simulink model "MIL_Visualisation"  (R2022b)
settings: Solver=VariableStepAuto  StartTime=0.0  StopTime=60  RelTol=1e-3
libraries: slpidlib x2, sim3dlib x1, sim3dautolib x1
settings Model: Creator=ok  LastModifiedBy=ok

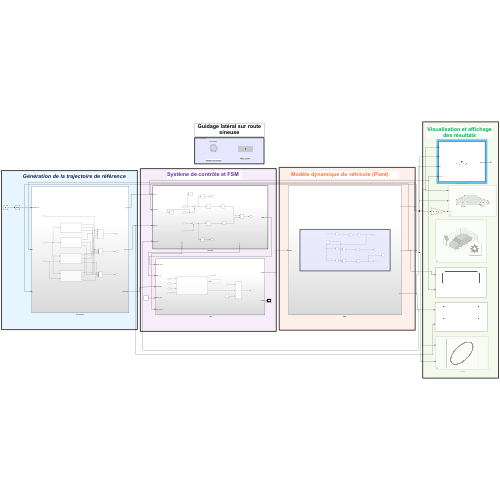
[thumbnail: Simulink's stored preview of the top-level diagram]
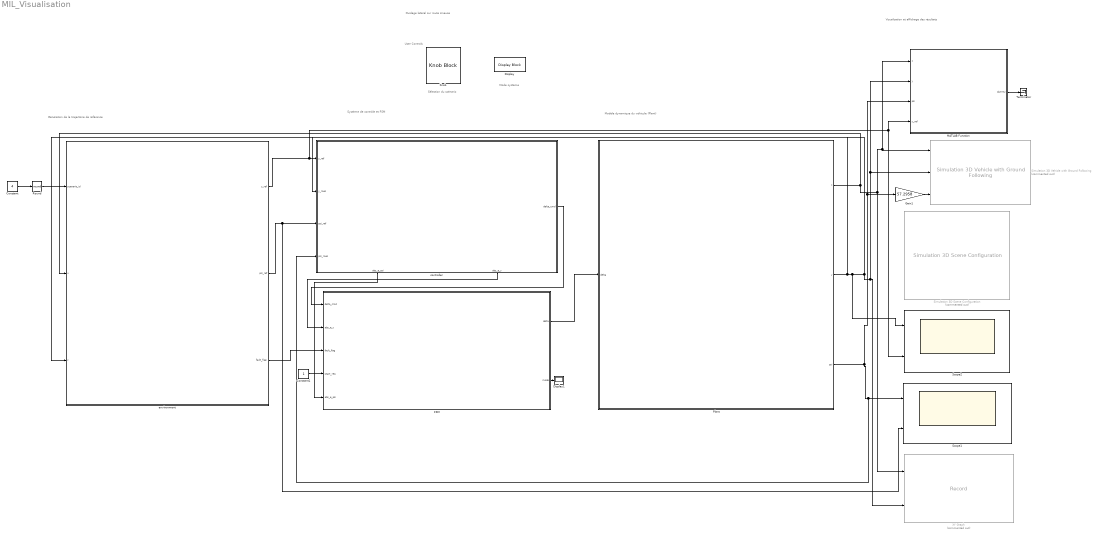
== system MIL_Visualisation ==
  note: Système de contrôle et FSM
  note: Génération de la trajectoire de référence
  note: Visualisation et affichage des résultats
  note: Sélection du scénario
  note: Mode système
  note: User Controls
  note: Modèle dynamique du véhicule (Plant)
  note: Guidage latéral sur route sineuse
  Constant : Constant  Value=4
  Constant1 : Constant
  Display : DisplayBlock  LabelPosition=Hide  Transparency=1
  Display1 : Display
  FSM : Subsystem
  Gain1 : Gain  Gain=57.2958
  Knob : KnobBlock  ScaleMin=1  ScaleMax=4  TickInterval=1
  MATLAB Function : MATLAB Function  TreatAsAtomicUnit=on
  "Plant " : Subsystem
  Round : Rounding  Operator=round
  Scope1 : Scope  NumInputPorts=2
  Scope2 : Scope  NumInputPorts=2
  Simulation 3D Scene Configuration : sim3dlib/Simulation 3D Scene Configuration  Priority=0  Commented=on  ProjectFormat=Default Scenes  SceneDesc=Straight road  ProjectName=C:\Program Files\MATLAB\R2022b\toolbox\shared\sim3d_projects\automotive_project\UE4\WindowsNoEditor\VehicleSimulation.exe  ScenePath=/Game/Maps/HwStrght  EnableOpenDRIVE=off  vehTagList={'Scene Origin';'SimulinkVehicle1'}  vehTag=Scene Origin  OpVisEn=off  Ts=1/60  EnableWindow=on  EnableRemoteAccess=off  EnableWeather=off  SunAltitude=40.0  SunAzimuth=90  clouds=10  wind=1  fog=0  rain=0  EnableGeospatial=off  OriginHeight=200  OriginLatitude=40.744652  OriginLongitude=-73.988864  MapStyle=Aerial  AdditionalAssetIDs=[]  UseAdvancedSunSky=off  SolarTime=11  TimeZone=-5  Day=21  Month=9  Year=2022  UseDaylightSavingTime=on  DSTStartDay=10  DSTStartMonth=3  DSTEndDay=3  DSTEndMonth=11  DSTSwitchHour=2  sensorTag=MainCamera1  sensorId=1  sensorName=MainCamera1  mountLoc=Origin  offsetFlag=off  tmountOffset=[0, 0, 0]  rmountOffset=[0, 0, 0]  HorizontalResolution=1280  VerticalResolution=720  HorizontalFOV=60  mountPoint=[0 0 0]  mountOrientation=[0 0 0]  aMode=3  ID=1  GeoTrigger=Inactive
      settings: LibrarySourceBlock=drivingsim3d/Simulation 3D Scene Configuration
  Simulation 3D Vehicle with Ground Following : sim3dautolib/Simulation 3D Vehicle with Ground Following  Priority=-1  Commented=on  PassVehMesh=Muscle car  MeshPath=/MathWorksAutomotiveContent/Vehicles/Muscle/Meshes/SK_MuscleCar.SK_MuscleCar  TrackWidth=1.9  WheelBase=3  WheelRadius=0.35  VehColor=Orange  InitialPos=[0, 0, 0]  InitialRot=[0, 0, 0]  ActorName=SimulinkVehicle1  SampleTime=-1  ActorType=SimulinkVehicle  ID=1  aMode=3  ActorTag=SimulinkVehicle1  CoordinateScheme=ISO  VehLightsControl=off  HeadlightColor=[ 1, 1, 1 ]  HighBeamIntensity=100000  LowBeamIntensity=60000  HighBeamConeAngle=70  LowBeamConeAngle=70  LeftHeadlightOrientation=[ 0, 0 ]  RightHeadlightOrientation=[ 0, 0 ]  BrakelightIntensity=500  ReverselightIntensity=500  SignallightIntensity=500  SignallightPeriod=1  SignalPulseWidth=50  TransformOutportEnabled=off
      settings: LibrarySourceBlock=drivingsim3d/Simulation 3D Vehicle with Ground Following
  Terminator : Terminator
  XY Graph : Record  Commented=on  FileSettingsInternal="{\"entries\":[{\"content\":{\"excelSettings\":{\"content\":{},\"type\":\"Streamout.ExcelSettings\"}},\"type\":\"Streamout.FileSettingStorage\",\"uuid\":\"06e8999a-84d6-4fbe-90db-6198f86497ce\"}],\"packageUris\":[\"http://schema.mathworks.com/mf0/streamout_blocks/R2020a\"],\"version\":\"1.0\"}"  Layout=[1 1]  SignalsInternal="{\"entries\":[{\"content\":{\"signals\":[{\"content\":{\"blockPath\":[\"testMIL/XY Graph\"],\"channel\":[],\"dimensions\":[1],\"domain\":\"testMIL/XY Graph\",\"lineColor\":\"#edb120\",\"plots\":[],\"port\":1,\"sid\":[],\"signalID\":1014,\"signalName\":\"Plant :1\"},\"type\":\"RecordBlkView.Signal\",\"uuid\":\"2eb3453d-083d-4465-a58f-0ec1d1455d5e\"},{\"content\":{\"blockPath\":[\"testMIL/XY Graph\"],\"channel\":[],\"dimensions\":[1],\"domain\":\"testMIL/XY Graph\",\"lineColor\":\"#7e2f8e\",\"plots\":[],\"port\":2,\"sid\":[],\"signalID\":1017,\"signalName\":\"Plant :2\"},\"type\":\"RecordBlkView.Signal\",\"uuid\":\"a053f1bc-5d23-4c0a-8de6-d9fee1b0b9c1\"}]},\"type\":\"RecordBlkView.InputSignals\",\"uuid\":\"f97cfab6-83bd-41ff-8d9c-43b8d98c9b4b\"}],\"packageUris\":[\"http://schema.mathworks.com/mf0/streamout_blocks/R2020a\"],\"version\":\"1.0\"}"  VisualizationBindings="{\"xyplotplugin\":{\"info\":[{\"series\":[],\"subplotID\":1}]}}"  CompatibilityTag=XY
  controller : Subsystem  TreatAsAtomicUnit=on
      settings: PortSchema="{\"entries\":[{\"content\":{\"sides\":[{\"content\":{\"connectorIds\":[\"In1\",\"In2\",\"In3\",\"In4\"]},\"type\":\"ConnectorPlacement.EquallySpacedRectSide\",\"uuid\":\"dce009df-b000-45c7-aa28-a3bb8a55b1fe\"},{\"content\":{\"connectorIds\":[\"Out1\"],\"side\":\"RIGHT\"},\"type\":\"ConnectorPlacement.EquallySpacedRectSide\",\"uuid\":\"27679ab1-5f7b-49ed-b0db-4270332b706f\"},{\"content\":{\"connectorIds\":[],\"side\":\"TOP\"},\"type\":\"ConnectorPlacement.EquallySpacedRectSide\",\"uuid\":\"474e0d2f-310b-4a94-af54-f468ed9e1b68\"},{\"content\":{\"connectorIds\":[\"Out2\",\"Out3\"],\"side\":\"BOTTOM\"},\"type\":\"ConnectorPlacement.EquallySpacedRectSide\",\"uuid\":\"e9194f37-6c87-4243-879e-6146eac92453\"}]},\"type\":\"ConnectorPlacement.EquallySpacedConnector\",\"uuid\":\"bf9faa3f-a673-4ccc-8b0a-d91001fa1506\"}],\"packageUris\":[\"http://schema.mathworks.com/mf0/Connector/R2020b\"],\"version\":\"1.0\"}"
  "environment " : Subsystem
  wires:
  "Plant "/1(x) -> XY Graph/1, Simulation 3D Vehicle with Ground Following/1, MATLAB Function/1(x), "environment "/2(x)
  controller/3(abs_e_y) -> FSM/2(abs_e_y)
  controller/2(abs_e_psi) -> FSM/5(abs_e_psi)
  "environment "/3(fault_flag) -> FSM/3(fault_flag)
  FSM/2(mode) -> Display1/1
  Constant/1 -> Round/1
  "Plant "/3(psi) -> controller/4(psi_mes), Scope1/1, Gain1/1, MATLAB Function/3(psi)
  "environment "/2(psi_ref) -> Scope1/2, controller/3(psi_ref)
  Round/1 -> "environment "/1(scenario_id)
  Constant1/1 -> FSM/4(start_req)
  FSM/1(delta) -> "Plant "/1(delta)
  "environment "/1(y_ref) -> MATLAB Function/4(y_ref), Scope2/2, controller/1(y_ref)
  MATLAB Function/1(dummy) -> Terminator/1
  "Plant "/2(y) -> controller/2(y_mes), Scope2/1, XY Graph/2, MATLAB Function/2(y), Simulation 3D Vehicle with Ground Following/2, "environment "/3(y)
  controller/1(delta_cmd) -> FSM/1(delta_cmd)
  Gain1/1 -> Simulation 3D Vehicle with Ground Following/3

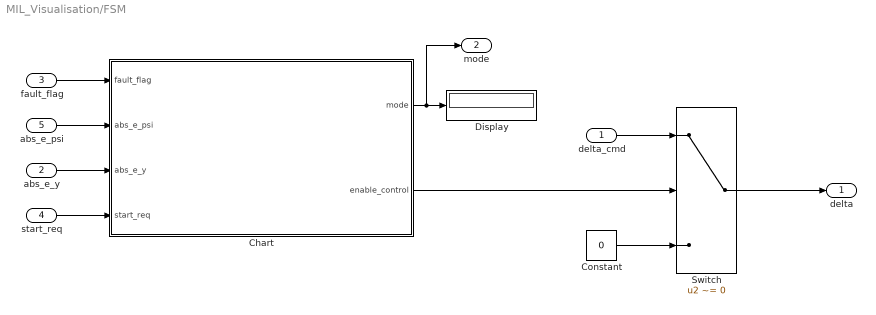
== system MIL_Visualisation/FSM ==
  delta_cmd : Inport
  abs_e_y : Inport  Port=2
  fault_flag : Inport  Port=3
  start_req : Inport  Port=4
  abs_e_psi : Inport  Port=5
  Chart : Stateflow chart  TreatAsAtomicUnit=on
  Constant : Constant  Value=0
  Display : Display
  Switch : Switch  Criteria=u2 ~= 0  SaturateOnIntegerOverflow=off  InputSameDT=off
  delta : Outport
  mode : Outport  Port=2
  wires:
  Chart/1(mode) -> mode/1, Display/1
  delta_cmd/1 -> Switch/1
  Switch/1 -> delta/1
  Chart/2(enable_control) -> Switch/2
  Constant/1 -> Switch/3
  abs_e_y/1 -> Chart/3(abs_e_y)
  fault_flag/1 -> Chart/1(fault_flag)
  abs_e_psi/1 -> Chart/2(abs_e_psi)
  start_req/1 -> Chart/4(start_req)

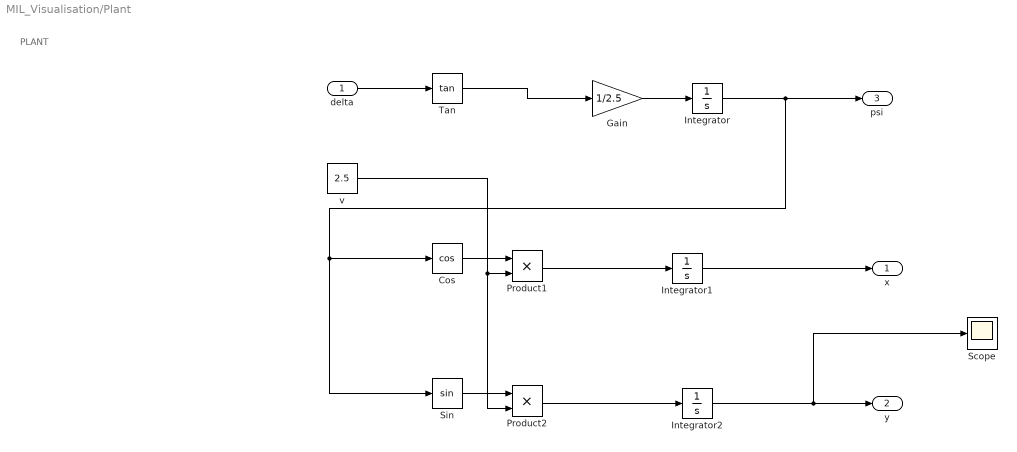
== system MIL_Visualisation/Plant  ==
  note: PLANT
  delta : Inport
  Cos : Trigonometry  Operator=cos
  Gain : Gain  Gain=1/2.5
  Integrator : Integrator
  Integrator1 : Integrator
  Integrator2 : Integrator
  Product1 : Product
  Product2 : Product
  Scope : Scope
  Sin : Trigonometry
  Tan : Trigonometry  Operator=tan
  v : Constant  Value=2.5
  x : Outport
  y : Outport  Port=2
  psi : Outport  Port=3
  wires:
  delta/1 -> Tan/1
  v/1 -> Product2/2, Product1/2
  Gain/1 -> Integrator/1
  Integrator/1 -> Sin/1, Cos/1, psi/1
  Cos/1 -> Product1/1
  Product1/1 -> Integrator1/1
  Integrator1/1 -> x/1
  Sin/1 -> Product2/1
  Product2/1 -> Integrator2/1
  Integrator2/1 -> Scope/1, y/1
  Tan/1 -> Gain/1

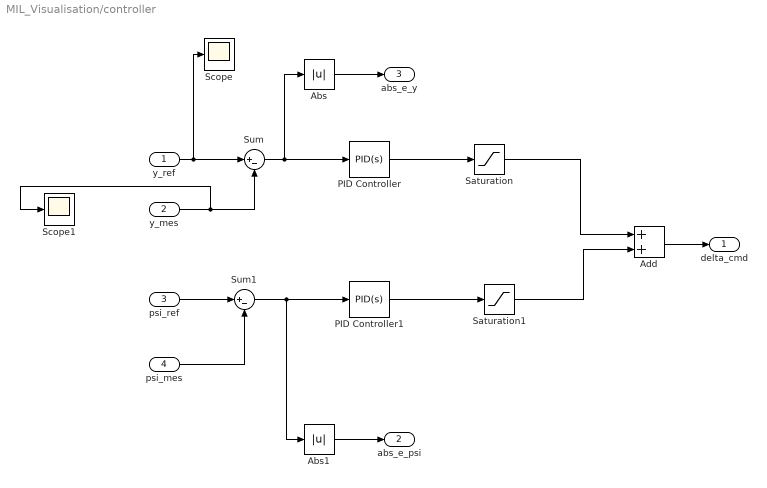
== system MIL_Visualisation/controller ==
  y_ref : Inport
  y_mes : Inport  Port=2
  psi_ref : Inport  Port=3
  psi_mes : Inport  Port=4
  Abs : Abs  SaturateOnIntegerOverflow=off
  Abs1 : Abs  SaturateOnIntegerOverflow=off
  Add : Sum
  PID Controller : slpidlib/PID Controller  Controller=PID  Form=Parallel  TimeDomain=Continuous-time  UseExternalTs=off  SampleTime=-1  IntegratorMethod=Forward Euler  FilterMethod=Forward Euler  ControllerParametersSource=internal  P=0.543076883773547  I=0.448698988285461  UseKiTs=off  D=0.162626525747815  N=212.929749678129  UseFilter=on  TunerSelectOption=Transfer Function Based (PID Tuner App)  InitialConditionSource=internal  InitialConditionForIntegrator=0  InitialConditionForFilter=0  DifferentiatorICPrevScaledInput=0  ExternalReset=none  TrackingMode=off  Kt=1  LimitOutput=off  SatLimitsSource=internal  UpperSaturationLimit=inf  LowerSaturationLimit=-inf  LinearizeAsGain=on  AntiWindupMode=none  Kb=1  LimitIntegrator=off  UpperIntegratorSaturationLimit=inf  LowerIntegratorSaturationLimit=-inf  POutMin=[]  POutMax=[]  IOutMin=[]  IOutMax=[]  DOutMin=[]  DOutMax=[]  NOutMin=[]  NOutMax=[]  SumOutMin=[]  SumOutMax=[]  SaturationOutMin=[]  SaturationOutMax=[]  PParamMin=[]  PParamMax=[]  IParamMin=[]  IParamMax=[]  DParamMin=[]  DParamMax=[]  NParamMin=[]  NParamMax=[]  KbParamMin=[]  KbParamMax=[]  KtParamMin=[]  KtParamMax=[]  KbOutMin=[]  KbOutMax=[]  KtOutMin=[]  KtOutMax=[]  IntegratorOutMin=[]  IntegratorOutMax=[]  FilterOutMin=[]  FilterOutMax=[]  SumI1OutMin=[]  SumI1OutMax=[]  SumI2OutMin=[]  SumI2OutMax=[]  SumI3OutMin=[]  SumI3OutMax=[]  SumI4OutMin=[]  SumI4OutMax=[]  SumDOutMin=[]  SumDOutMax=[]  DifferentiatorOutMin=[]  DifferentiatorOutMax=[]  FilterDiffOutCoefMin=[]  FilterDiffOutCoefMax=[]  ReciprocalOutMin=[]  ReciprocalOutMax=[]  SumDenOutMin=[]  SumDenOutMax=[]  SumNumOutMin=[]  SumNumOutMax=[]  DivideOutMin=[]  DivideOutMax=[]  UdiffTsProdOutMin=[]  UdiffTsProdOutMax=[]  NTsProdOutMin=[]  NTsProdOutMax=[]  UintegralTsProdOutMin=[]  UintegralTsProdOutMax=[]  UngainTsProdOutMin=[]  UngainTsProdOutMax=[]  ClampingZeroOutDataTypeStr=Inherit: Inherit via back propagation  ClampingZeroOutMin=[]  ClampingZeroOutMax=[]  FilterDenConstantOutDataTypeStr=Inherit: Inherit via back propagation  FilterDenConstantOutMin=[]  FilterDenConstantOutMax=[]  PCopyOutDataTypeStr=Inherit: Inherit via back propagation  PCopyOutMin=[]  PCopyOutMax=[]  NCopyOutDataTypeStr=Inherit: Inherit via back propagation  NCopyOutMin=[]  NCopyOutMax=[]  IntegratorContinuousStateAttributes=''  IntegratorStateMustResolveToSignalObject=off  IntegratorRTWStateStorageClass=Auto  FilterContinuousStateAttributes=''  FilterStateMustResolveToSignalObject=off  FilterRTWStateStorageClass=Auto  ParallelPVariant=InternalParameters  IdealPVariant=Disabled  IVariant=InternalParameters  DVariant=InternalParameters  IntegratorVariant=Continuous  SatVariant=Disabled  AWVariant=Passthrough  PCopyVariant=Disabled  TRVariant=Disabled  FdbkBlocksVariant=Forward  IdealPFdbkVariant=Disabled  SatFdbkVariant=Disabled  DerivativeFilterVariant=ContFilter  NVariant=InternalParameters  NCopyVariant=Disabled  FilterICVariant=InternalICsFilter  IntegratorICVariant=InternalICs  ExternalResetVariant=Disabled  TRSumVariant=Passthrough  SumFdbkVariant=Disabled  SumVariant=Sum_PID  TsampFilterVariant=InternalTs  TsampNgainVariant=Passthrough  TsampIntegralVariant=Passthrough  ExternalSaturationOutDataTypeStr=Inherit: Same as second input
  PID Controller1 : slpidlib/PID Controller  Controller=PID  Form=Parallel  TimeDomain=Continuous-time  UseExternalTs=off  SampleTime=-1  IntegratorMethod=Forward Euler  FilterMethod=Forward Euler  ControllerParametersSource=internal  P=68.8464008350311  I=1387.43622401745  UseKiTs=off  D=-0.169418101050233  N=123.850290878266  UseFilter=on  TunerSelectOption=Transfer Function Based (PID Tuner App)  InitialConditionSource=internal  InitialConditionForIntegrator=0  InitialConditionForFilter=0  DifferentiatorICPrevScaledInput=0  ExternalReset=none  TrackingMode=off  Kt=1  LimitOutput=off  SatLimitsSource=internal  UpperSaturationLimit=inf  LowerSaturationLimit=-inf  LinearizeAsGain=on  AntiWindupMode=none  Kb=1  LimitIntegrator=off  UpperIntegratorSaturationLimit=inf  LowerIntegratorSaturationLimit=-inf  POutMin=[]  POutMax=[]  IOutMin=[]  IOutMax=[]  DOutMin=[]  DOutMax=[]  NOutMin=[]  NOutMax=[]  SumOutMin=[]  SumOutMax=[]  SaturationOutMin=[]  SaturationOutMax=[]  PParamMin=[]  PParamMax=[]  IParamMin=[]  IParamMax=[]  DParamMin=[]  DParamMax=[]  NParamMin=[]  NParamMax=[]  KbParamMin=[]  KbParamMax=[]  KtParamMin=[]  KtParamMax=[]  KbOutMin=[]  KbOutMax=[]  KtOutMin=[]  KtOutMax=[]  IntegratorOutMin=[]  IntegratorOutMax=[]  FilterOutMin=[]  FilterOutMax=[]  SumI1OutMin=[]  SumI1OutMax=[]  SumI2OutMin=[]  SumI2OutMax=[]  SumI3OutMin=[]  SumI3OutMax=[]  SumI4OutMin=[]  SumI4OutMax=[]  SumDOutMin=[]  SumDOutMax=[]  DifferentiatorOutMin=[]  DifferentiatorOutMax=[]  FilterDiffOutCoefMin=[]  FilterDiffOutCoefMax=[]  ReciprocalOutMin=[]  ReciprocalOutMax=[]  SumDenOutMin=[]  SumDenOutMax=[]  SumNumOutMin=[]  SumNumOutMax=[]  DivideOutMin=[]  DivideOutMax=[]  UdiffTsProdOutMin=[]  UdiffTsProdOutMax=[]  NTsProdOutMin=[]  NTsProdOutMax=[]  UintegralTsProdOutMin=[]  UintegralTsProdOutMax=[]  UngainTsProdOutMin=[]  UngainTsProdOutMax=[]  ClampingZeroOutDataTypeStr=Inherit: Inherit via back propagation  ClampingZeroOutMin=[]  ClampingZeroOutMax=[]  FilterDenConstantOutDataTypeStr=Inherit: Inherit via back propagation  FilterDenConstantOutMin=[]  FilterDenConstantOutMax=[]  PCopyOutDataTypeStr=Inherit: Inherit via back propagation  PCopyOutMin=[]  PCopyOutMax=[]  NCopyOutDataTypeStr=Inherit: Inherit via back propagation  NCopyOutMin=[]  NCopyOutMax=[]  IntegratorContinuousStateAttributes=''  IntegratorStateMustResolveToSignalObject=off  IntegratorRTWStateStorageClass=Auto  FilterContinuousStateAttributes=''  FilterStateMustResolveToSignalObject=off  FilterRTWStateStorageClass=Auto  ParallelPVariant=InternalParameters  IdealPVariant=Disabled  IVariant=InternalParameters  DVariant=InternalParameters  IntegratorVariant=Continuous  SatVariant=Disabled  AWVariant=Passthrough  PCopyVariant=Disabled  TRVariant=Disabled  FdbkBlocksVariant=Forward  IdealPFdbkVariant=Disabled  SatFdbkVariant=Disabled  DerivativeFilterVariant=ContFilter  NVariant=InternalParameters  NCopyVariant=Disabled  FilterICVariant=InternalICsFilter  IntegratorICVariant=InternalICs  ExternalResetVariant=Disabled  TRSumVariant=Passthrough  SumFdbkVariant=Disabled  SumVariant=Sum_PID  TsampFilterVariant=InternalTs  TsampNgainVariant=Passthrough  TsampIntegralVariant=Passthrough  ExternalSaturationOutDataTypeStr=Inherit: Same as second input
  Saturation : Saturate
  Saturation1 : Saturate
  Scope : Scope
  Scope1 : Scope
  Sum : Sum  Inputs=|+-
  Sum1 : Sum  Inputs=|+-
  delta_cmd : Outport
  abs_e_psi : Outport  Port=2
  abs_e_y : Outport  Port=3
  wires:
  y_ref/1 -> Scope/1, Sum/1
  y_mes/1 -> Scope1/1, Sum/2
  Sum/1 -> PID Controller/1, Abs/1
  psi_ref/1 -> Sum1/1
  psi_mes/1 -> Sum1/2
  PID Controller/1 -> Saturation/1
  Sum1/1 -> Abs1/1, PID Controller1/1
  PID Controller1/1 -> Saturation1/1
  Add/1 -> delta_cmd/1
  Saturation/1 -> Add/1
  Saturation1/1 -> Add/2
  Abs/1 -> abs_e_y/1
  Abs1/1 -> abs_e_psi/1

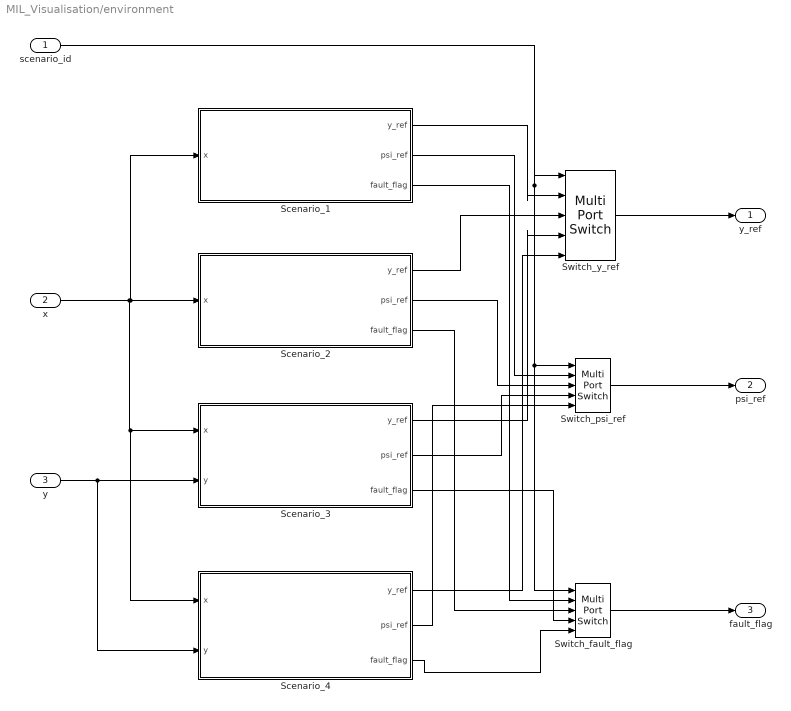
== system MIL_Visualisation/environment  ==
  scenario_id : Inport
  x : Inport  Port=2
  y : Inport  Port=3
  Scenario_1 : Subsystem
  Scenario_2 : Subsystem
  Scenario_3 : Subsystem
  Scenario_4 : Subsystem
  Switch_fault_flag : MultiPortSwitch  Inputs=4  SaturateOnIntegerOverflow=off  InputSameDT=off
  Switch_psi_ref : MultiPortSwitch  Inputs=4  SaturateOnIntegerOverflow=off  InputSameDT=off
  Switch_y_ref : MultiPortSwitch  Inputs=4  SaturateOnIntegerOverflow=off  InputSameDT=off
  y_ref : Outport
  psi_ref : Outport  Port=2
  fault_flag : Outport  Port=3
  wires:
  scenario_id/1 -> Switch_fault_flag/1, Switch_psi_ref/1, Switch_y_ref/1
  Scenario_1/1(y_ref) -> Switch_y_ref/2
  Scenario_2/1("y_ref ") -> Switch_y_ref/3
  Scenario_3/1("y_ref ") -> Switch_y_ref/4
  Scenario_4/1(y_ref) -> Switch_y_ref/5
  Scenario_1/2(psi_ref) -> Switch_psi_ref/2
  Scenario_2/2("psi_ref ") -> Switch_psi_ref/3
  Scenario_3/2("psi_ref ") -> Switch_psi_ref/4
  Scenario_4/2(psi_ref) -> Switch_psi_ref/5
  Scenario_1/3(fault_flag) -> Switch_fault_flag/2
  Scenario_2/3(fault_flag) -> Switch_fault_flag/3
  Scenario_3/3(fault_flag) -> Switch_fault_flag/4
  Scenario_4/3(fault_flag) -> Switch_fault_flag/5
  Switch_fault_flag/1 -> fault_flag/1
  Switch_psi_ref/1 -> psi_ref/1
  Switch_y_ref/1 -> y_ref/1
  x/1 -> Scenario_4/1(x), Scenario_3/1(x), Scenario_1/1(x), Scenario_2/1(x)
  y/1 -> Scenario_4/2(y), Scenario_3/2(y)

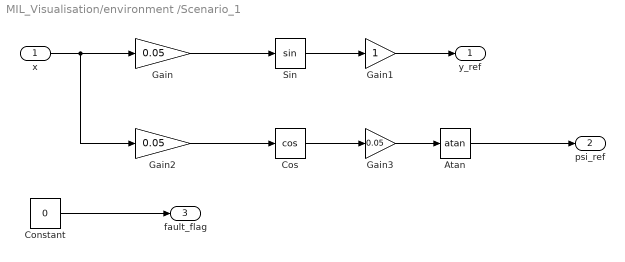
== system MIL_Visualisation/environment /Scenario_1 ==
  x : Inport
  Atan : Trigonometry  Operator=atan
  Constant : Constant  Value=0
  Cos : Trigonometry  Operator=cos
  Gain : Gain  Gain=0.05
  Gain1 : Gain
  Gain2 : Gain  Gain=0.05
  Gain3 : Gain  Gain=0.05
  Sin : Trigonometry
  y_ref : Outport
  psi_ref : Outport  Port=2
  fault_flag : Outport  Port=3
  wires:
  x/1 -> Gain2/1, Gain/1
  Gain/1 -> Sin/1
  Sin/1 -> Gain1/1
  Gain1/1 -> y_ref/1
  Cos/1 -> Gain3/1
  Gain2/1 -> Cos/1
  Gain3/1 -> Atan/1
  Atan/1 -> psi_ref/1
  Constant/1 -> fault_flag/1

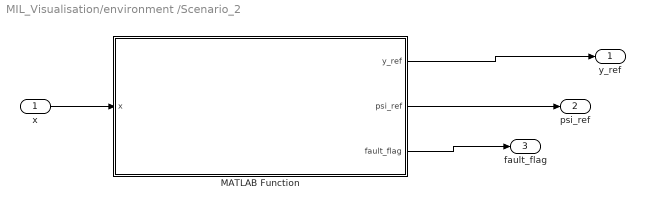
== system MIL_Visualisation/environment /Scenario_2 ==
  x : Inport
  MATLAB Function : MATLAB Function  TreatAsAtomicUnit=on
  "y_ref " : Outport
  "psi_ref " : Outport  Port=2
  fault_flag : Outport  Port=3
  wires:
  MATLAB Function/1(y_ref) -> "y_ref "/1
  MATLAB Function/2(psi_ref) -> "psi_ref "/1
  MATLAB Function/3(fault_flag) -> fault_flag/1
  x/1 -> MATLAB Function/1(x)

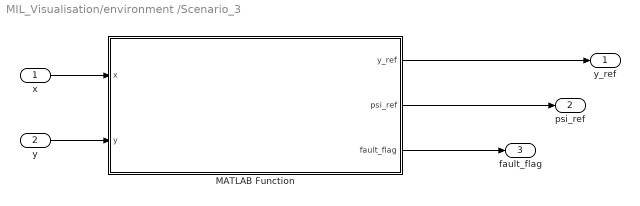
== system MIL_Visualisation/environment /Scenario_3 ==
  x : Inport
  y : Inport  Port=2
  MATLAB Function : MATLAB Function  TreatAsAtomicUnit=on
  "y_ref " : Outport
  "psi_ref " : Outport  Port=2
  fault_flag : Outport  Port=3
  wires:
  MATLAB Function/1(y_ref) -> "y_ref "/1
  MATLAB Function/3(fault_flag) -> fault_flag/1
  y/1 -> MATLAB Function/2(y)
  MATLAB Function/2(psi_ref) -> "psi_ref "/1
  x/1 -> MATLAB Function/1(x)

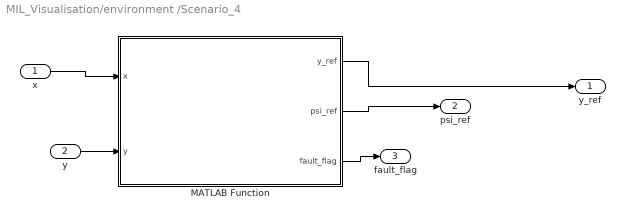
== system MIL_Visualisation/environment /Scenario_4 ==
  x : Inport
  y : Inport  Port=2
  MATLAB Function : MATLAB Function  TreatAsAtomicUnit=on
  y_ref : Outport
  psi_ref : Outport  Port=2
  fault_flag : Outport  Port=3
  wires:
  x/1 -> MATLAB Function/1(x)
  MATLAB Function/1(y_ref) -> y_ref/1
  MATLAB Function/2(psi_ref) -> psi_ref/1
  MATLAB Function/3(fault_flag) -> fault_flag/1
  y/1 -> MATLAB Function/2(y)

== matlab function MIL_Visualisation/environment /Scenario_3/MATLAB Function ==
  data: x input; y_ref output; y input; psi_ref output; fault_flag output
function [y_ref, psi_ref, fault_flag] = scenario3_onecurve(x, y)
%#codegen

% Paramètres de la route
A = 2.0;      % amplitude de la courbe
xc = 25.0;    % centre de la courbe
sigma = 6.0;  % largeur de la courbe

% Référence latérale : une seule bosse douce
dx = x - xc;
y_ref = A * exp(-(dx*dx)/(2*sigma*sigma));

% Dérivée par rapport à x
dy_dx = y_ref * ( -dx / (sigma*sigma) );

% Orientation de référence
psi_ref = atan(dy_dx);

% Pas de défaut dans ce scénario
fault_flag = 0;

== matlab function MIL_Visualisation/environment /Scenario_2/MATLAB Function ==
  data: x input; y_ref output; psi_ref output; fault_flag output
function [y_ref, psi_ref, fault_flag] = environment_fun(x)
%#codegen

% Route sinueuse simple et cohérente
A = 2;       % amplitude
B = 0.1;     % fréquence spatiale

y_ref = A*sin(B*x);

% pente de la route
dy_dx = A*B*cos(B*x);

% orientation de la route
psi_ref = atan(dy_dx);

% défaut
fault_flag = 0;

end

== stateflow chart MIL_Visualisation/FSM/Chart ==
  state Init
    en:
    enable_control = 0;
    mode = 0;
  state Nominal
    en:
    enable_control = 1;
    mode = 2;
  state Standby
    en:
    enable_control = 0;
    mode = 1;
  state Emergency
    en:
    enable_control = 0;
    mode = 3;
  (default) -> Init
  Standby -> Nominal : [start_req == 1 && fault_flag == 0]
  Init -> Standby : after(0.5,sec)
  Emergency -> Standby : [start_req == 0 && fault_flag == 0]
  Nominal -> Emergency : [fault_flag == 1 || abs_e_y > 1.5 || abs_e_psi > 0.5]
  data: mode output; enable_control output; fault_flag input; abs_e_psi input; abs_e_y input; start_req input

== matlab function MIL_Visualisation/MATLAB Function ==
  settings: updateMethod=DISCRETE
  data: x input; dummy output; y input; psi input; y_ref input
function dummy = draw_vehicle_2D(x, y, psi, y_ref)
%#codegen

coder.extrinsic('figure','clf','hold','grid','xlabel','ylabel', ...
                'title','legend','plot','fill','set','xlim','ylim', ...
                'drawnow','gca','gcf')

persistent hTraj hRef hCar Xveh Yveh Xref Yref isInit ax fig

dummy = 0;

if isempty(isInit)
    fig = figure(20);
    clf(fig);

    % Grande fenêtre
    set(fig,'Units','normalized');
    set(fig,'Position',[0.08 0.08 0.84 0.82]);

    ax = gca;
    hold(ax,'on');
    grid(ax,'on');

    % IMPORTANT : ne pas mettre axis equal
    set(ax,'Units','normalized');
    set(ax,'Position',[0.06 0.10 0.90 0.82]);

    xlabel(ax,'X [m]','FontSize',14);
    ylabel(ax,'Y [m]','FontSize',14);
    title(ax,'Suivi 2D du vehicule sur route','FontSize',16,'FontWeight','bold');

    % Rouge d'abord
    hTraj = plot(ax,0,0,'r-','LineWidth',2);

    % Bleu ensuite pour qu'il soit au-dessus
    hRef  = plot(ax,0,0,'b--o', ...
        'LineWidth',3, ...
        'MarkerSize',4, ...
        'MarkerFaceColor','b');

    % Rectangle véhicule
    hCar  = fill(ax,0,0,'r','EdgeColor','k','LineWidth',1.5);

    legend(ax, ...
        'Trajectoire reelle', ...
        'Route de reference', ...
        'Vehicule', ...
        'Location','northwest');

    Xveh = [];
    Yveh = [];
    Xref = [];
    Yref = [];

    isInit = true;
end

% Historique
Xveh = [Xveh, x];
Yveh = [Yveh, y];

Xref = [Xref, x];
Yref = [Yref, y_ref];

% Mise à jour courbes
set(hTraj,'XData',Xveh,'YData',Yveh);
set(hRef ,'XData',Xref,'YData',Yref);

% Rectangle du véhicule
L = 3.0;
W = 1.6;

corners = [ L/2,  W/2;
            L/2, -W/2;
           -L/2, -W/2;
           -L/2,  W/2]';

R = [cos(psi) -sin(psi);
     sin(psi)  cos(psi)];

rot = R * corners;

Xcar = rot(1,:) + x;
Ycar = rot(2,:) + y;

set(hCar,'XData',Xcar,'YData',Ycar);

% Axes qui remplissent bien la fenêtre
xmin = min([Xveh Xref]);
xmax = max([Xveh Xref]);

if isempty(xmin) || isempty(xmax)
    xmin = 0;
    xmax = 10;
end

if (xmax - xmin) < 40
    xc = 0.5*(xmin + xmax);
    xmin = xc - 20;
    xmax = xc + 20;
end

ymin = min([Yveh Yref]);
ymax = max([Yveh Yref]);

if isempty(ymin) || isempty(ymax)
    ymin = -5;
    ymax = 5;
end

if (ymax - ymin) < 12
    yc = 0.5*(ymin + ymax);
    ymin = yc - 6;
    ymax = yc + 6;
else
    ymin = ymin - 1;
    ymax = ymax + 1;
end

xlim(ax,[xmin xmax]);
ylim(ax,[ymin ymax]);

drawnow;

== matlab function MIL_Visualisation/environment /Scenario_4/MATLAB Function ==
  data: x input; y_ref output; psi_ref output; fault_flag output; y input
function [y_ref, psi_ref, fault_flag] = scenario4_simple(x, y)
%#codegen
% Scenario 4 : sinusoide puis virage

A = 2;        % amplitude sinusoide
B = 0.08;     % frequence
x_turn = 60;  % point ou on tourne

if x < x_turn
    
    % ===== PARTIE 1 : SINUSOIDE =====
    y_ref = A * sin(B*x);
    dy_dx = A * B * cos(B*x);

else
    
    % ===== PARTIE 2 : VIRAGE CLAIR =====
    R = 20;   % rayon du virage
    
    dx = x - x_turn;
    
    % courbe type parabole (simple et stable)
    y_ref = A * sin(B*x_turn) + (dx^2)/(2*R);
    
    dy_dx = dx / R;

end

% orientation
psi_ref = atan(dy_dx);

% pas de defaut
fault_flag = 0;
